simulink library "CH_Library"  (R2021a)
settings: Solver=VariableStepAuto  StartTime=0.0  StopTime=10.0  RelTol=1e-3
undefined symbols (not defined in the file or in its folder): params, X, Y, Z
libraries: sm_lib x116, nesl_utility x53, $bdroot x20, sm_humanoid_walker_lib x13, fl_lib x10, simulink x8, ee_lib x3, simulink_extras x1
(part 1 of 4)
settings Model: Creator=The MathWorks, Inc.  LastModifiedBy=coa19cdd
settings SolverCC: AlgebraicLoopSolver=TrustRegion
settings DebuggingCC: SFMachineParentedDataDiag=warning

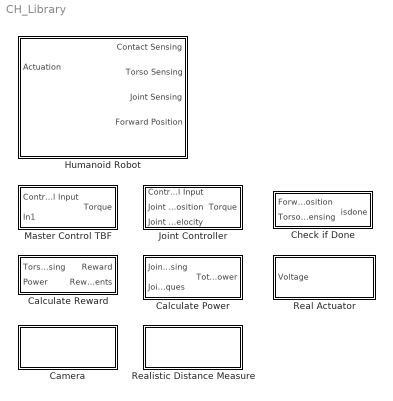
== system CH_Library ==
  Calculate Power : Subsystem
  Calculate Reward : Subsystem  mask{forwardReward=params.reward.forwardRewardWeight, timestepReward=params.reward.timestepRewardWeight, powerPenalty=params.reward.powerPenaltyWeight, verticalPenalty=params.reward.verticalPenaltyWeight, lateralPenalty=params.reward.lateralPenaltyWeight}
      mask prompts: forwardReward "Forward velcoity reward scaling"; timestepReward "Timestep reward scaling"; powerPenalty "Power penalty scaling"; verticalPenalty "Vertical displacement penalty scaling"; lateralPenalty "Lateral displacement penalty scaling"
  Camera : Subsystem  mask{X_ROT=0, Z_ROT=0, X_TF=0, Y_TF=0, Z_TF=0}
      mask prompts: X_ROT "X rotation Value"; Z_ROT "Z Rotation Value"; X_TF "X Displacement"; Y_TF "Y Displacement"; Z_TF "Z Displacement"
      mask DialogControl Container7 Prompt: Camera Rotation
      mask DialogControl Container8 Prompt: Camera Transform
  Check if Done : Subsystem  mask{verticalStop=params.stoppingCriteria.heightChange, lateralStop=params.stoppingCriteria.lateral, angularStop=params.stoppingCriteria.angle, timeoutTime=params.stoppingCriteria.timeoutTime, timeoutDistance=params.stoppingCriteria.timeoutDistance}
      mask prompts: verticalStop "Vertical Displacement Stopping Criteria (m)"; lateralStop "Lateral Displacement Stopping Criteria (m)"; angularStop "Rotation Stopping Criteria (deg)"; timeoutTime "Timeout Time"; timeoutDistance "Timeout Distance"
  Humanoid Robot : Subsystem  mask{contactRadius=params.contact.contactRadius, contactStiffness=params.contact.stiffness, contactDamping=params.contact.damping, contactTWidth=params.contact.transitionWidth, contactStaticFriction=params.contact.staticFriction, contactDynamicFriction=params.contact.dynamicFriction, contactCriticalVelocity=params.contact.criticalVelocity, footDensity=params.materialProperties.lowerBodyDensity, lowerLegDensity=params.materialProperties.lowerBodyDensity, upperLegDensity=params.materialProperties.lowerBodyDensity, hipDensity=params.materialProperties.lowerBodyDensity, trunkDensity=params.materialProperties.upperBodyDensity, shoulderDensity=params.materialProperties.upperBodyDensity, upperArmDensity=params.materialProperties.upperBodyDensity, lowerArmDensity=params.materialProperties.upperBodyDensity, handDensity=params.materialProperties.upperBodyDensity, headDensity=params.materialProperties.upperBodyDensity, hipUpperLimit=params.jointLimits.hipFrontalUpperLimit, hipLowerLimit=params.jointLimits.hipFrontalLowerLimit, kneeUpperLimit=params.jointLimits.kneeUpperLimit, kneeLowerLimit=params.jointLimits.kneeLowerLimit, ankleUpperLimit=params.jointLimits.ankleUpperLimit, ankleLowerLimit=params.jointLimits.ankleLowerLimit, shoulderFrontalUpperLimit=params.jointLimits.shoulderFrontalUpperLimit, shoulderFrontalLowerLimit=params.jointLimits.shoulderFrontalLowerLimit, shoulderSagittalUpperLimit=params.jointLimits.shoulderSagittalUpperLimit, shoulderSagittalLowerLimit=params.jointLimits.shoulderSagittalLowerLimit, elbowUpperLimit=params.jointLimits.ankleUpperLimit, elbowLowerLimit=params.jointLimits.shoulderSagittalLowerLimit, wristUpperLimit=params.jointLimits.ankleUpperLimit, wristLowerLimit=params.jointLimits.shoulderSagittalLowerLimit}
      mask prompts: contactRadius "Contact Sphere Radius (m)"; contactStiffness "Contact Stiffness (N/m)"; contactDamping "Contact Damping (Ns/m)"; contactTWidth "Contact Tranisiton Region Width (m)"; contactStaticFriction "Contact Static Friction"; contactDynamicFriction "Contact Dynamic Friction"; contactCriticalVelocity "Contact Critical Velocity (m/s)"; footDensity "Foot Density (kg/m^3)"; lowerLegDensity "Lower Leg Density (kg/m^3)"; upperLegDensity "Upper Leg Density (kg/m^3)"; hipDensity "Hip Density (kg/m^3)"; trunkDensity "Trunk Density (kg/m^3)"; shoulderDensity "Shoulder Density (kg/m^3)"; upperArmDensity "Upper Arm Density (kg/m^3)"; lowerArmDensity "Lower Arm Density (kg/m^3)"; handDensity "Hand Density (kg/m^3)"; headDensity "Neck / Head Density (kg/m^3)"; hipUpperLimit "Hip Frontal Upper Limit (deg)"; hipLowerLimit "Hip Frontal Lower Limit (deg)"; kneeUpperLimit "Knee Upper Limit (deg)"; kneeLowerLimit "Knee Lower Limit (deg)"; ankleUpperLimit "Ankle Upper Limit (deg)"; ankleLowerLimit "Ankle Lower Limit (deg)"; shoulderFrontalUpperLimit "Shoulder Frontal Upper Limit (deg)"; shoulderFrontalLowerLimit "Shoulder Frontal Lower Limit (deg)"; shoulderSagittalUpperLimit "Shoulder Sagittal Upper Limit (deg)"; shoulderSagittalLowerLimit "Shoulder Sagittal Lower Limit (deg)"; elbowUpperLimit "Elbow Upper Limit (deg)"; elbowLowerLimit "Elbow Lower Limit (deg)"; wristUpperLimit "Wrist Upper Limit (deg)"; wristLowerLimit "Wrist Lower Limit (deg)"
      mask DialogControl Container4 Prompt: Contact Parameters
      mask DialogControl Container9 Prompt: Material Properties
      mask DialogControl Container12 Prompt: Joint Parameters
      mask DialogControl Container10 Prompt: LegLimits
      mask DialogControl Container11 Prompt: ArmLimits
  Joint Controller : Subsystem  mask{jointStiffness=0, jointDamping=0, jointUpperLimit=0, jointLowerLimit=0, jointTorqueLimit=0}
      mask prompts: jointStiffness "Joint Control Stiffness (N*m/rad)"; jointDamping "Joint Control Damping (N*m*s/rad)"; jointUpperLimit "Joint Upper Limit (deg)"; jointLowerLimit "Joint Lower Limt (deg)"; jointTorqueLimit "Joint Absolute Torque Limit (N*m)"
      mask DialogControl DescTextVar Prompt: Stiffness based joint controller.
  Master Control TBF : Subsystem
  Real Actuator : Subsystem  mask{ArmatureInductance=0, StallTorque=0, NoLoadSpeed=0, RatedDCSupply=0, gearRatio=5.0}
      mask prompts: ArmatureInductance "Armature Inductance"; StallTorque "Stall Torque"; NoLoadSpeed "Maximum Speed"; RatedDCSupply "Rated DC Supply Voltage"; gearRatio "Gearing ratio"
      settings: PortSchema="{\"entries\":[{\"content\":{\"sides\":[{\"content\":{\"connectorIds\":[\"In1\"]},\"type\":\"ConnectorPlacement.EquallySpacedRectSide\",\"uuid\":\"1974e72c-7cd0-4a5e-a369-6bd8d81aeaf4\"},{\"content\":{\"connectorIds\":[],\"side\":\"RIGHT\"},\"type\":\"ConnectorPlacement.EquallySpacedRectSide\",\"uuid\":\"85686b63-5bbe-4355-a058-7d010135ed1d\"},{\"content\":{\"connectorIds\":[\"LConn1\",\"LConn2\"],\"side\":\"TOP\"},\"type\":\"ConnectorPlacement.EquallySpacedRectSide\",\"uuid\":\"5bc14ff2-42d4-4faf-9552-836511591ac4\"}]},\"type\":\"ConnectorPlacement.EquallySpacedConnector\",\"uuid\":\"9c3e7e84-92ff-47c5-b2ae-92b3c6517a43\"}],\"packageUris\":[\"http://schema.mathworks.com/mf0/Connector/R2020b\"],\"version\":\"1.0\"}"
      mask DialogControl Container4 Prompt: Motor parameters
      mask DialogControl Container5 Prompt: Gearbox Ratio
  Realistic Distance Measure : Subsystem  mask{LEDC=0.500}
      mask prompts: LEDC "LED Current"

== system CH_Library/Calculate Power ==
  Joint Sensing : Inport
  Joint Torques : Inport  Port=2
  Bus Selector1 : BusSelector  OutputSignals=LegSense.RightLegSense.RHFS.rhThetaDot,LegSense.RightLegSense.RHSS.rhssThetaDot,LegSense.RightLegSense.RKS.rkThetaDot,LegSense.RightLegSense.RAS.raThetaDot,LegSense.RightLegSense.RASS.lasThetaDot,LegSense.LeftLegSense.LHFS.lhThetaDot,LegSense.LeftLegSense.LHSS.lhsThetaDot,LegSense.LeftLegSense.LKS.lkThetaDot,LegSense.LeftLegSense.LASS.lasThetaDot,LegSense.LeftLegSense.LAS.laThetaDot,ArmSense.RightArmSense.RSFS.rsfThetaDot,ArmSense.RightArmSense.RSSS.rssThetaDot,ArmSense.RightArmSense.RES.reThetaDot,ArmSense.RightArmSense.RWS.rwThetaDot,ArmSense.LeftArmSense.LSFS.lsfThetaDot,ArmSense.LeftArmSense.LSSS.lssThetaDot,ArmSense.LeftArmSense.LES.leThetaDot,ArmSense.LeftArmSense.LWS.lwThetaDot
  Mux : Mux  Inputs=18
  Product : Product
  Sum of Elements : Sum  Inputs=+
  Unit Delay : UnitDelay  SampleTime=-1  HasFrameUpgradeWarning=on
  Total Power : Outport
  wires:
  Bus Selector1/18 -> Mux/18  "<lwThetaDot>"
  Bus Selector1/17 -> Mux/17  "<leThetaDot>"
  Bus Selector1/16 -> Mux/16  "<lssThetaDot>"
  Bus Selector1/15 -> Mux/15  "<lsfThetaDot>"
  Bus Selector1/14 -> Mux/14  "<rwThetaDot>"
  Bus Selector1/13 -> Mux/13  "<reThetaDot>"
  Bus Selector1/12 -> Mux/12  "<rssThetaDot>"
  Bus Selector1/11 -> Mux/11  "<rsfThetaDot>"
  Bus Selector1/10 -> Mux/10  "<laThetaDot>"
  Bus Selector1/9 -> Mux/9  "<lasThetaDot>"
  Bus Selector1/8 -> Mux/8  "<lkThetaDot>"
  Bus Selector1/7 -> Mux/7  "<lhsThetaDot>"
  Bus Selector1/6 -> Mux/6  "<lhThetaDot>"
  Bus Selector1/5 -> Mux/5  "<lasThetaDot>"
  Bus Selector1/4 -> Mux/4  "<raThetaDot>"
  Bus Selector1/3 -> Mux/3  "<rkThetaDot>"
  Bus Selector1/2 -> Mux/2  "<rhssThetaDot>"
  Bus Selector1/1 -> Mux/1  "<rhThetaDot>"
  Product/1 -> Sum of Elements/1
  Joint Sensing/1 -> Bus Selector1/1
  Mux/1 -> Product/1
  Joint Torques/1 -> Product/2
  Sum of Elements/1 -> Unit Delay/1
  Unit Delay/1 -> Total Power/1

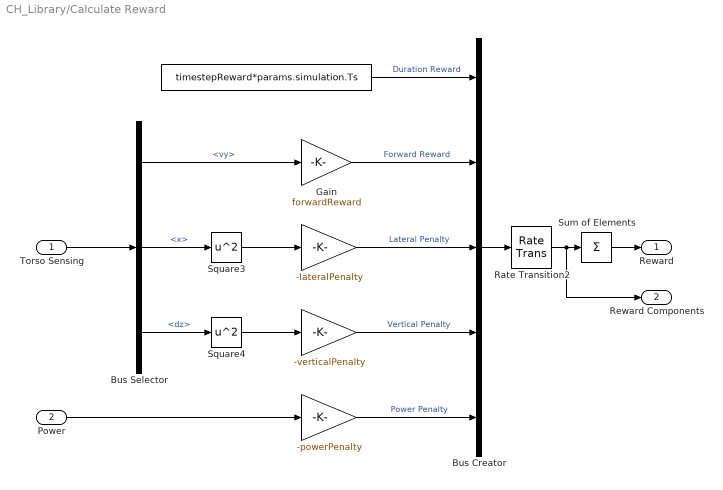
== system CH_Library/Calculate Reward ==
  Torso Sensing : Inport
  Power : Inport  Port=2
  " " : Gain  Gain=-lateralPenalty
  "     " : Gain  Gain=-verticalPenalty
  "                    " : Gain  Gain=-powerPenalty
  "                       " : Constant  Value=timestepReward*params.simulation.Ts
  Bus Creator : BusCreator  Inputs=5
  Bus Selector : BusSelector  OutputSignals=signal2.vy,signal2.x,signal2.dz
  Gain : Gain  Gain=forwardReward
  Rate Transition2 : RateTransition  OutPortSampleTime=params.simulation.Ts
  Square3 : Math  Operator=square  SignedPower=on  SaturateOnIntegerOverflow=on
  Square4 : Math  Operator=square  SignedPower=on  SaturateOnIntegerOverflow=on
  Sum of Elements : Sum  Inputs=+
  Reward : Outport  VectorParamsAs1DForOutWhenUnconnected=off
  Reward Components : Outport  Port=2  VectorParamsAs1DForOutWhenUnconnected=off
  wires:
  Torso Sensing/1 -> Bus Selector/1
  Power/1 -> "                    "/1
  Square4/1 -> "     "/1
  Bus Selector/3 -> Square4/1  "<dz>"
  Square3/1 -> " "/1
  Bus Selector/2 -> Square3/1  "<x>"
  Sum of Elements/1 -> Reward/1
  " "/1 -> Bus Creator/3  "Lateral Penalty"
  "                    "/1 -> Bus Creator/5  "Power Penalty"
  "                       "/1 -> Bus Creator/1  "Duration Reward"
  Bus Selector/1 -> Gain/1  "<vy>"
  Gain/1 -> Bus Creator/2  "Forward Reward"
  "     "/1 -> Bus Creator/4  "Vertical Penalty"
  Bus Creator/1 -> Rate Transition2/1
  Rate Transition2/1 -> Reward Components/1, Sum of Elements/1

== system CH_Library/Camera ==
  Camera Location : sm_lib/Frames and Transforms/Rigid Transform  TranslationMethod=Cartesian  TranslationStandardOffset=0  TranslationLengthUnit=m  TranslationStandardAxis=+Z  TranslationCartesianOffset=[X_TF Y_TF Z_TF]  TranslationROffset=0  TranslationROffsetUnits=m  TranslationZOffset=0  TranslationZOffsetUnits=m  TranslationThetaOffset=0  TranslationThetaOffsetUnits=deg  RotationMethod=None  RotationAngleUnits=deg  RotationStandardAxis=+Z  RotationAngle=0.0  RotationArbitraryAxis=[0 0 1]  FollAlignAxisA=+X  BaseAlignAxisA=+Y  FollAlignAxisB=+Y  BaseAlignAxisB=+Z  RotationSequenceAxes=FollowerAxes  RotationSequence=XYX  RotationSequenceAngles=[0 0 0]  RotationSequenceAnglesUnits=deg  RotationMatrix=[1 0 0; 0 1 0; 0 0 1]
  Camera Rotation : sm_lib/Frames and Transforms/Rigid Transform  TranslationMethod=None  TranslationStandardOffset=0  TranslationLengthUnit=m  TranslationStandardAxis=+Z  TranslationCartesianOffset=[0 0 0]  TranslationROffset=0  TranslationROffsetUnits=m  TranslationZOffset=0  TranslationZOffsetUnits=m  TranslationThetaOffset=0  TranslationThetaOffsetUnits=deg  RotationMethod=RotationSequence  RotationAngleUnits=deg  RotationStandardAxis=+Z  RotationAngle=0.0  RotationArbitraryAxis=[0 0 1]  FollAlignAxisA=+X  BaseAlignAxisA=+Y  FollAlignAxisB=+Y  BaseAlignAxisB=+Z  RotationSequenceAxes=FollowerAxes  RotationSequence=ZXZ  RotationSequenceAngles=[Z_ROT X_ROT 0]  RotationSequenceAnglesUnits=deg  RotationMatrix=[1 0 0; 0 1 0; 0 0 1]
  Spherical Solid : sm_lib/Body Elements/Spherical Solid  GraphicAmbientColor=[0.15 0.15 0.15 1.0]  BasedOnType=Density  CenterOfMass=[0 0 0]  CenterOfMassUnits=m  GraphicDiffuseColor=[0.2 1.0 0.2]  Density=1000  DensityUnits=kg/m^3  DoExposeReferenceFrame=on  GraphicEmissiveColor=[0.0 0.0 0.0 1.0]  ExportEntireGeometry=off  SerializedExposedGeometries=<ExposedGeometries/>  SerializedFrames=<Frames/>  MarkerShape=Sphere  MarkerSize=10  GraphicType=FromGeometry  InertiaType=PointMass  Mass=1  MassUnits=g  MomentsOfInertia=[1 1 1]  MomentsOfInertiaUnits=kg*m^2  GraphicOpacity=1.0  ProductsOfInertia=[0 0 0]  ProductsOfInertiaUnits=kg*m^2  GraphicShininess=75  GraphicSpecularColor=[0.5 0.5 0.5 1.0]  SphereRadius=0.01  SphereRadiusUnits=m  GraphicVisPropType=SimpleVisualProperties
  Camera : PMIOPort  Side=Right
  connections:
  Spherical Solid/RConn1 -- Camera Location/RConn1
  Camera Rotation/RConn1 -- Camera Location/LConn1
  Camera/RConn1 -- Camera Rotation/LConn1

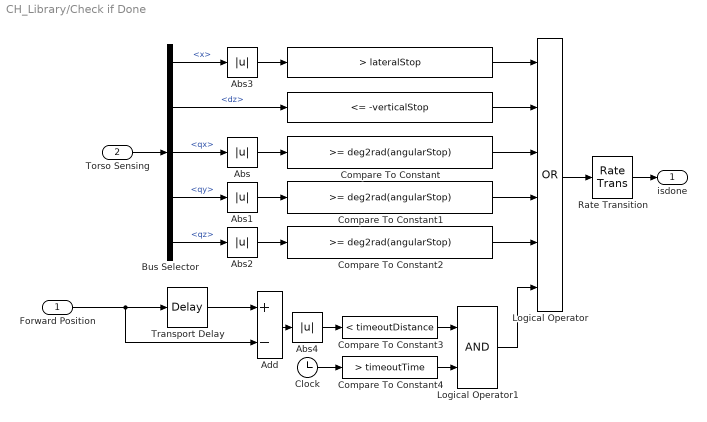
== system CH_Library/Check if Done ==
  Forward Position : Inport
  Torso Sensing : Inport  Port=2
  " " : simulink/Logic and Bit Operations/Compare To Constant  relop=<=  const=-verticalStop  OutDataTypeStr=boolean  ZeroCross=off
  "             " : simulink/Logic and Bit Operations/Compare To Constant  relop=>  const=lateralStop  OutDataTypeStr=boolean
  Abs{,1..3} (4 alike) : Abs  ZeroCross=off
  Abs4 : Abs
  Add : Sum  Inputs=+-
  Bus Selector : BusSelector  OutputSignals=signal2.x,signal2.dz,signal1.qx,signal1.qy,signal1.qz
  Clock : Clock
  Compare To Constant : simulink/Logic and Bit Operations/Compare To Constant  relop=>=  const=deg2rad(angularStop)  OutDataTypeStr=boolean  ZeroCross=off
  Compare To Constant1 : simulink/Logic and Bit Operations/Compare To Constant  relop=>=  const=deg2rad(angularStop)  OutDataTypeStr=boolean  ZeroCross=off
  Compare To Constant2 : simulink/Logic and Bit Operations/Compare To Constant  relop=>=  const=deg2rad(angularStop)  OutDataTypeStr=boolean  ZeroCross=off
  Compare To Constant3 : simulink/Logic and Bit Operations/Compare To Constant  relop=<  const=timeoutDistance  OutDataTypeStr=boolean
  Compare To Constant4 : simulink/Logic and Bit Operations/Compare To Constant  relop=>  const=timeoutTime  OutDataTypeStr=boolean
  Logical Operator : Logic  Operator=OR  Inputs=6  AllPortsSameDT=off  OutDataTypeStr=boolean
  Logical Operator1 : Logic  AllPortsSameDT=off  OutDataTypeStr=boolean
  Rate Transition : RateTransition  OutPortSampleTime=params.simulation.Ts
  Transport Delay : TransportDelay  DelayTime=timeoutTime  BufferSize=8192
  isdone : Outport  VectorParamsAs1DForOutWhenUnconnected=off
  wires:
  Bus Selector/2 -> " "/1  "<dz>"
  Torso Sensing/1 -> Bus Selector/1
  " "/1 -> Logical Operator/2
  Bus Selector/3 -> Abs/1  "<qx>"
  Bus Selector/4 -> Abs1/1  "<qy>"
  Compare To Constant/1 -> Logical Operator/3
  Abs/1 -> Compare To Constant/1
  Abs1/1 -> Compare To Constant1/1
  Logical Operator/1 -> Rate Transition/1
  Abs3/1 -> "             "/1
  Bus Selector/1 -> Abs3/1  "<x>"
  "             "/1 -> Logical Operator/1
  Abs2/1 -> Compare To Constant2/1
  Bus Selector/5 -> Abs2/1  "<qz>"
  Compare To Constant2/1 -> Logical Operator/5
  Compare To Constant1/1 -> Logical Operator/4
  Rate Transition/1 -> isdone/1
  Forward Position/1 -> Add/2, Transport Delay/1
  Transport Delay/1 -> Add/1
  Add/1 -> Abs4/1
  Abs4/1 -> Compare To Constant3/1
  Clock/1 -> Compare To Constant4/1
  Logical Operator1/1 -> Logical Operator/6
  Compare To Constant3/1 -> Logical Operator1/1
  Compare To Constant4/1 -> Logical Operator1/2

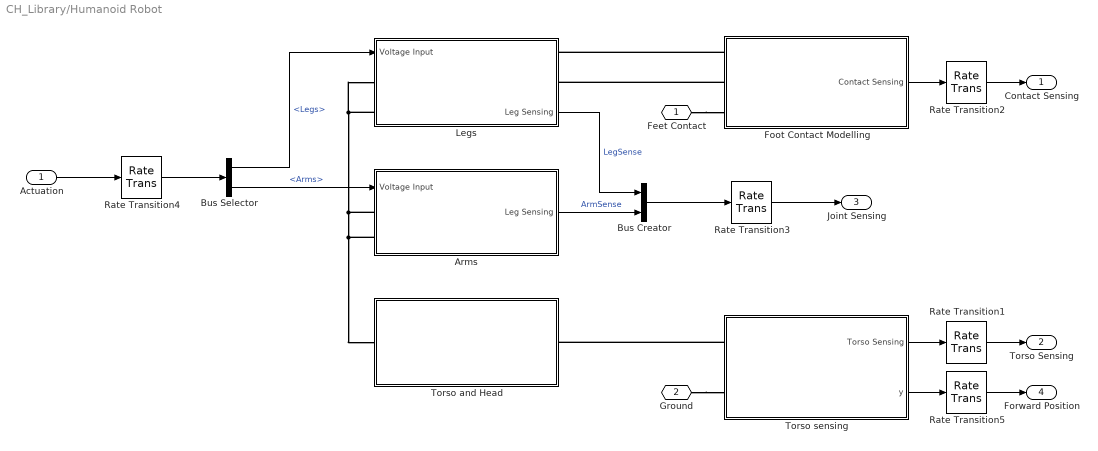
== system CH_Library/Humanoid Robot ==
  Actuation : Inport
  Arms : Subsystem
  Bus Creator : BusCreator  Inputs=2
  Bus Selector : BusSelector  OutputSignals=Legs,Arms
  Foot Contact Modelling : Subsystem
  Legs : Subsystem
      settings: PortSchema="{\"entries\":[{\"content\":{\"sides\":[{\"content\":{\"connectorIds\":[\"In1\",\"LConn1\",\"LConn2\"]},\"type\":\"ConnectorPlacement.EquallySpacedRectSide\",\"uuid\":\"23351413-746b-4a06-be1b-12a3513cfbfe\"},{\"content\":{\"connectorIds\":[\"RConn1\",\"RConn2\",\"Out1\"],\"side\":\"RIGHT\"},\"type\":\"ConnectorPlacement.EquallySpacedRectSide\",\"uuid\":\"11cf50da-2174-4e1a-8294-03a32c066ee9\"},{\"content\":{\"connectorIds\":[],\"side\":\"TOP\"},\"type\":\"ConnectorPlacement.EquallySpacedRectSide\",\"uuid\":\"131464a5-eb41-49e4-a10b-6e29adf56ddb\"}]},\"type\":\"ConnectorPlacement.EquallySpacedConnector\",\"uuid\":\"d1829b9e-a701-4b79-9220-5146acc6850e\"}],\"packageUris\":[\"http://schema.mathworks.com/mf0/Connector/R2020b\"],\"version\":\"1.0\"}"
  Rate Transition{1..5} (5 alike) : RateTransition  OutPortSampleTime=params.simulation.Ts
  Torso and Head : Subsystem
  Torso sensing : Subsystem
  Feet Contact : PMIOPort  Side=Right
  " Ground" : PMIOPort  Port=2  Side=Left
  Contact Sensing : Outport
  Torso Sensing : Outport  Port=2
  Joint Sensing : Outport  Port=3
  Forward Position : Outport  Port=4
  wires:
  Foot Contact Modelling/1(Contact Sensing) -> Rate Transition2/1
  Actuation/1 -> Rate Transition4/1
  Torso sensing/1(Torso Sensing) -> Rate Transition1/1
  Rate Transition2/1 -> Contact Sensing/1
  Rate Transition1/1 -> Torso Sensing/1
  Rate Transition3/1 -> Joint Sensing/1
  Rate Transition5/1 -> Forward Position/1
  Torso sensing/2(y) -> Rate Transition5/1
  Rate Transition4/1 -> Bus Selector/1
  Bus Selector/1 -> Legs/1(Voltage Input)  "<Legs>"
  Bus Selector/2 -> Arms/1(Voltage Input)  "<Arms>"
  Bus Creator/1 -> Rate Transition3/1
  Legs/1(Leg Sensing) -> Bus Creator/1  "LegSense"
  Arms/1(Leg Sensing) -> Bus Creator/2  "ArmSense"
  connections:
  Legs/LConn2 -- Legs/LConn1 -- Arms/LConn1 -- Arms/LConn2 -- Torso and Head/LConn1
  Torso sensing/LConn1 -- Torso and Head/RConn1
  Feet Contact/RConn1 -- Foot Contact Modelling/LConn3
  Foot Contact Modelling/LConn1 -- Legs/RConn1
  Foot Contact Modelling/LConn2 -- Legs/RConn2
  " Ground"/RConn1 -- Torso sensing/LConn2

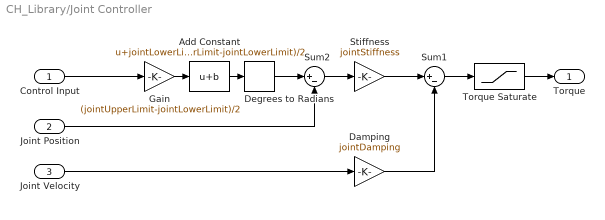
== system CH_Library/Joint Controller ==
  Control Input : Inport
  Joint Position : Inport  Port=2
  Joint Velocity : Inport  Port=3
  Add Constant : Bias  Bias=jointLowerLimit + (jointUpperLimit-jointLowerLimit)/2
  Damping : Gain  Gain=jointDamping
  Degrees to Radians : simulink_extras/Transformations/Degrees to Radians
  Gain : Gain  Gain=(jointUpperLimit-jointLowerLimit)/2
  Stiffness : Gain  Gain=jointStiffness
  Sum1 : Sum  Inputs=|+-
  Sum2 : Sum  Inputs=|+-
  Torque Saturate : Saturate  UpperLimit=jointTorqueLimit  LowerLimit=-jointTorqueLimit  ZeroCross=off
  Torque : Outport
  wires:
  Damping/1 -> Sum1/2
  Stiffness/1 -> Sum1/1
  Add Constant/1 -> Degrees to Radians/1
  Gain/1 -> Add Constant/1
  Control Input/1 -> Gain/1
  Sum2/1 -> Stiffness/1
  Joint Velocity/1 -> Damping/1
  Sum1/1 -> Torque Saturate/1
  Torque Saturate/1 -> Torque/1
  Degrees to Radians/1 -> Sum2/1
  Joint Position/1 -> Sum2/2

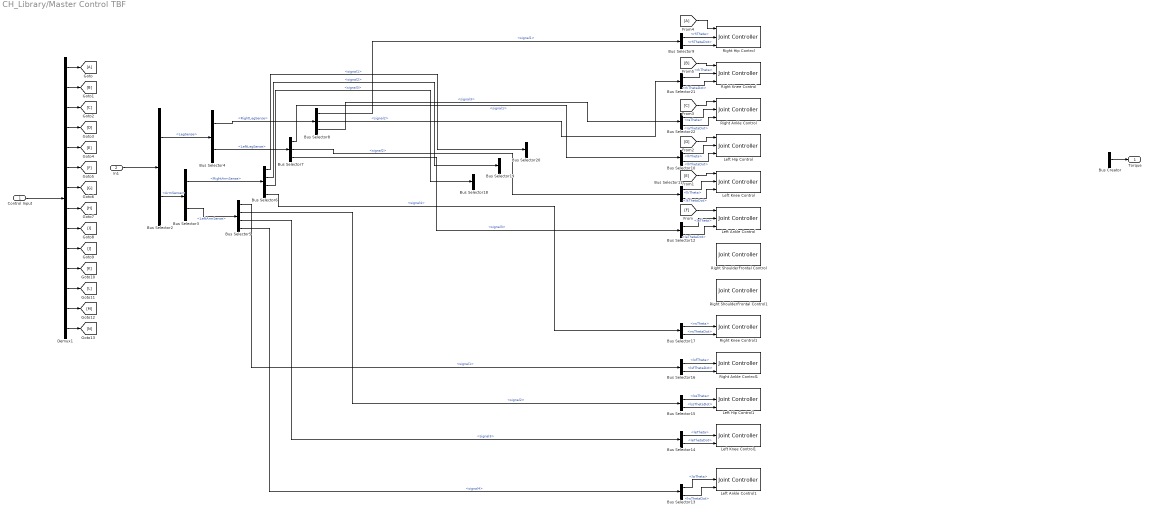
== system CH_Library/Master Control TBF ==
  Control Input : Inport
  In1 : Inport  Port=2
  Bus Creator : BusCreator  Inputs=2
  Bus Selector10 : BusSelector  OutputSignals=lhTheta,lhThetaDot
  Bus Selector11 : BusSelector  OutputSignals=lkTheta,lkThetaDot
  Bus Selector12 : BusSelector  OutputSignals=laTheta,laThetaDot
  Bus Selector13 : BusSelector  OutputSignals=lwTheta,lwThetaDot
  Bus Selector14 : BusSelector  OutputSignals=leTheta,leThetaDot
  Bus Selector15 : BusSelector  OutputSignals=lssTheta,lssThetaDot
  Bus Selector16 : BusSelector  OutputSignals=lsfTheta,lsfThetaDot
  Bus Selector17 : BusSelector  OutputSignals=rwTheta,rwThetaDot
  Bus Selector18 : BusSelector  OutputSignals=reTheta,reThetaDot
  Bus Selector19 : BusSelector  OutputSignals=rssTheta,rssThetaDot
  Bus Selector2 : BusSelector  OutputSignals=LegSense,ArmSense
  Bus Selector20 : BusSelector  OutputSignals=rsfTheta,rsfThetaDot
  Bus Selector21 : BusSelector  OutputSignals=rkTheta,rkThetaDot
  Bus Selector22 : BusSelector  OutputSignals=raTheta,raThetaDot
  Bus Selector3 : BusSelector  OutputSignals=RightArmSense,LeftArmSense
  Bus Selector4 : BusSelector  OutputSignals=RightLegSense,LeftLegSense
  Bus Selector5 : BusSelector  OutputSignals=signal1,signal2,signal3,signal4
  Bus Selector6 : BusSelector  OutputSignals=signal1,signal2,signal3,signal4
  Bus Selector7 : BusSelector  OutputSignals=signal1,signal2,signal3
  Bus Selector8 : BusSelector  OutputSignals=signal1,signal2,signal3
  Bus Selector9 : BusSelector  OutputSignals=rhTheta,rhThetaDot
  Demux1 : Demux  Outputs=14
  Left Ankle Control : sm_humanoid_walker_lib/Joint Controller  jointStiffness=params.controller.ankleStiffness  jointDamping=params.controller.ankleDamping  jointUpperLimit=params.jointLimits.ankleUpperLimit  jointLowerLimit=params.jointLimits.ankleLowerLimit  jointTorqueLimit=params.torqueLimits.ankle
  Left Ankle Control1 : sm_humanoid_walker_lib/Joint Controller  jointStiffness=params.controller.ankleStiffness  jointDamping=params.controller.ankleDamping  jointUpperLimit=params.jointLimits.ankleUpperLimit  jointLowerLimit=params.jointLimits.ankleLowerLimit  jointTorqueLimit=params.torqueLimits.ankle
  Left Hip Control : sm_humanoid_walker_lib/Joint Controller  jointStiffness=params.controller.hipFrontalStiffness  jointDamping=params.controller.hipFrontalDamping  jointUpperLimit=params.jointLimits.hipFrontalUpperLimit  jointLowerLimit=params.jointLimits.hipFrontalLowerLimit  jointTorqueLimit=params.torqueLimits.hipFrontal
  Left Hip Control1 : sm_humanoid_walker_lib/Joint Controller  jointStiffness=params.controller.hipFrontalStiffness  jointDamping=params.controller.hipFrontalDamping  jointUpperLimit=params.jointLimits.hipFrontalUpperLimit  jointLowerLimit=params.jointLimits.hipFrontalLowerLimit  jointTorqueLimit=params.torqueLimits.hipFrontal
  Left Knee Control : sm_humanoid_walker_lib/Joint Controller  jointStiffness=params.controller.kneeStiffness  jointDamping=params.controller.kneeDamping  jointUpperLimit=params.jointLimits.kneeUpperLimit  jointLowerLimit=params.jointLimits.kneeLowerLimit  jointTorqueLimit=params.torqueLimits.knee
  Left Knee Control1 : sm_humanoid_walker_lib/Joint Controller  jointStiffness=params.controller.kneeStiffness  jointDamping=params.controller.kneeDamping  jointUpperLimit=params.jointLimits.kneeUpperLimit  jointLowerLimit=params.jointLimits.kneeLowerLimit  jointTorqueLimit=params.torqueLimits.knee
  Right Ankle Control : sm_humanoid_walker_lib/Joint Controller  jointStiffness=params.controller.ankleStiffness  jointDamping=params.controller.ankleDamping  jointUpperLimit=params.jointLimits.ankleUpperLimit  jointLowerLimit=params.jointLimits.ankleLowerLimit  jointTorqueLimit=params.torqueLimits.ankle
  Right Ankle Control1 : sm_humanoid_walker_lib/Joint Controller  jointStiffness=params.controller.ankleStiffness  jointDamping=params.controller.ankleDamping  jointUpperLimit=params.jointLimits.ankleUpperLimit  jointLowerLimit=params.jointLimits.ankleLowerLimit  jointTorqueLimit=params.torqueLimits.ankle
  Right Hip Control : sm_humanoid_walker_lib/Joint Controller  jointStiffness=params.controller.hipFrontalStiffness  jointDamping=params.controller.hipFrontalDamping  jointUpperLimit=params.jointLimits.hipFrontalUpperLimit  jointLowerLimit=params.jointLimits.hipFrontalLowerLimit  jointTorqueLimit=params.torqueLimits.hipFrontal
  Right Knee Control : sm_humanoid_walker_lib/Joint Controller  jointStiffness=params.controller.kneeStiffness  jointDamping=params.controller.kneeDamping  jointUpperLimit=params.jointLimits.kneeUpperLimit  jointLowerLimit=params.jointLimits.kneeLowerLimit  jointTorqueLimit=params.torqueLimits.knee
  Right Knee Control1 : sm_humanoid_walker_lib/Joint Controller  jointStiffness=params.controller.kneeStiffness  jointDamping=params.controller.kneeDamping  jointUpperLimit=params.jointLimits.kneeUpperLimit  jointLowerLimit=params.jointLimits.kneeLowerLimit  jointTorqueLimit=params.torqueLimits.knee
  Right ShoulderFrontal Control : sm_humanoid_walker_lib/Joint Controller  jointStiffness=params.controller.hipFrontalStiffness  jointDamping=params.controller.hipFrontalDamping  jointUpperLimit=params.jointLimits.shoulderFrontalUpperLimit  jointLowerLimit=params.jointLimits.shoulderFrontalLowerLimit  jointTorqueLimit=params.torqueLimits.hipFrontal
  Right ShoulderFrontal Control1 : sm_humanoid_walker_lib/Joint Controller  jointStiffness=params.controller.hipFrontalStiffness  jointDamping=params.controller.hipFrontalDamping  jointUpperLimit=params.jointLimits.shoulderFrontalUpperLimit  jointLowerLimit=params.jointLimits.shoulderFrontalLowerLimit  jointTorqueLimit=params.torqueLimits.hipFrontal
  Torque : Outport
  wires:
  Control Input/1 -> Demux1/1
  Demux1/1 -> [A]
  Demux1/6 -> [F]
  Demux1/5 -> [E]
  Demux1/4 -> [D]
  Demux1/3 -> [C]
  Demux1/2 -> [B]
  [F] -> Left Ankle Control/1
  [E] -> Left Knee Control/1
  [D] -> Left Hip Control/1
  [C] -> Right Ankle Control/1
  [B] -> Right Knee Control/1
  Demux1/7 -> [G]
  Demux1/8 -> [H]
  Demux1/9 -> [I]
  Demux1/10 -> [J]
  Demux1/11 -> [K]
  Demux1/12 -> [L]
  Bus Creator/1 -> Torque/1
  ? -> Bus Creator/1
  Demux1/13 -> [M]
  Demux1/14 -> [N]
  Bus Selector7/2 -> Bus Selector11/1  "<signal2>"
  Bus Selector6/1 -> Bus Selector20/1  "<signal1>"
  Bus Selector4/2 -> Bus Selector7/1  "<LeftLegSense>"
  Bus Selector8/3 -> Bus Selector22/1  "<signal3>"
  Bus Selector8/1 -> Bus Selector9/1  "<signal1>"
  Bus Selector3/1 -> Bus Selector6/1  "<RightArmSense>"
  Bus Selector2/2 -> Bus Selector3/1  "<ArmSense>"
  Bus Selector7/1 -> Bus Selector10/1  "<signal1>"
  Bus Selector7/3 -> Bus Selector12/1  "<signal3>"
  In1/1 -> Bus Selector2/1
  Bus Selector8/2 -> Bus Selector21/1  "<signal2>"
  Bus Selector4/1 -> Bus Selector8/1  "<RightLegSense>"
  Bus Selector5/3 -> Bus Selector14/1  "<signal3>"
  Bus Selector6/2 -> Bus Selector19/1  "<signal2>"
  Bus Selector3/2 -> Bus Selector5/1  "<LeftArmSense>"
  Bus Selector5/4 -> Bus Selector13/1  "<signal4>"
  Bus Selector5/1 -> Bus Selector16/1  "<signal1>"
  Bus Selector6/4 -> Bus Selector17/1  "<signal4>"
  Bus Selector5/2 -> Bus Selector15/1  "<signal2>"
  Bus Selector6/3 -> Bus Selector18/1  "<signal3>"
  Bus Selector2/1 -> Bus Selector4/1  "<LegSense>"
  Bus Selector9/1 -> Right Hip Control/2  "<rhTheta>"
  Bus Selector9/2 -> Right Hip Control/3  "<rhThetaDot>"
  [A] -> Right Hip Control/1
  Bus Selector21/1 -> Right Knee Control/2  "<rkTheta>"
  Bus Selector21/2 -> Right Knee Control/3  "<rkThetaDot>"
  Bus Selector22/1 -> Right Ankle Control/2  "<raTheta>"
  Bus Selector22/2 -> Right Ankle Control/3  "<raThetaDot>"
  Bus Selector10/1 -> Left Hip Control/2  "<lhTheta>"
  Bus Selector10/2 -> Left Hip Control/3  "<lhThetaDot>"
  Bus Selector11/1 -> Left Knee Control/2  "<lkTheta>"
  Bus Selector11/2 -> Left Knee Control/3  "<lkThetaDot>"
  Bus Selector12/1 -> Left Ankle Control/2  "<laTheta>"
  Bus Selector12/2 -> Left Ankle Control/3  "<laThetaDot>"
  Bus Selector13/2 -> Left Ankle Control1/3  "<lwThetaDot>"
  Bus Selector13/1 -> Left Ankle Control1/2  "<lwTheta>"
  Bus Selector14/1 -> Left Knee Control1/2  "<leTheta>"
  Bus Selector14/2 -> Left Knee Control1/3  "<leThetaDot>"
  Bus Selector15/2 -> Left Hip Control1/3  "<lssThetaDot>"
  Bus Selector15/1 -> Left Hip Control1/2  "<lssTheta>"
  Bus Selector16/1 -> Right Ankle Control1/2  "<lsfTheta>"
  Bus Selector16/2 -> Right Ankle Control1/3  "<lsfThetaDot>"
  Bus Selector17/2 -> Right Knee Control1/3  "<rwThetaDot>"
  Bus Selector17/1 -> Right Knee Control1/2  "<rwTheta>"

== system CH_Library/Real Actuator ==
  Voltage : Inport
  Controlled Voltage Source : fl_lib/Electrical/Electrical Sources/Controlled Voltage Source
  DC Motor : ee_lib/Electromechanical/Brushed Motors/DC Motor  field_option=ee.enum.field_option.pm  Rf=100 Ohm  Lf=1 H  Laf=0.15 H  If0=0 A  parameterization=ee.enum.dcparam_option.torque_speed  Ra=3.9 Ohm  La=ArmatureInductance H  emf_or_torque=ee.enum.emf_or_torque.ki  Kv=0.072e-3 V/rpm  Ki=6.876e-4 N*m/A  T_stall=StallTorque N*m  w_max="NoLoadSpeed   rpm"  w_rated=15000 rpm  P_rated=0.08 W  V_rated=RatedDCSupply V  J=0.01 g*cm^2  lam_param=ee.enum.lam_param.damping  lam=0 N*m/(rad/s)  i_noload=0 A  V_i_noload=1.5 V  speed0=0 rpm  enable_fault_armature=ee.enum.faults.faultEnable.no  rev_faulted=1 / 3  G_faulted_armature=1e-5 S  fault_trigger_armature=ee.enum.faults.faultTrigger.behavioral  t_fault_armature=1 s  max_permissible_current_armature=4 A  t_fail_on_current_armature=1 s  enable_fault_field=ee.enum.faults.faultEnable.no  G_faulted_field=1e-5 S  fault_trigger_field=ee.enum.faults.faultTrigger.temporal  t_fault_field=1 s  max_permissible_current_field=inf A  t_fail_on_current_field=1 s  fault_action=ee.enum.faults.faultAction.none  alpha=3.93e-3 1/K  Tmeas=25 degC  thermal_mass=100 J/K  initial_temperature=25 degC
  Electrical Reference : fl_lib/Electrical/Electrical Elements/Electrical Reference
  Gear Box : fl_lib/Mechanical/Mechanisms/Gear Box  ratio=gearRatio  t_in_specify=off  t_in_priority=None  t_in=0 N*m  t_in_nominal_specify=off  t_in_nominal_unit=N*m  t_in_nominal_value=1  t_out_specify=off  t_out_priority=None  t_out=0 N*m  t_out_nominal_specify=off  t_out_nominal_unit=N*m  t_out_nominal_value=1
  Mechanical Rotational Reference : fl_lib/Mechanical/Rotational Elements/Mechanical Rotational Reference
  Rotational Multibody Interface1 : fl_lib/Mechanical/Multibody Interfaces/Rotational Multibody Interface
      settings: SourceProductBaseCode=SS
  Simulink-PS Converter : nesl_utility/Simulink-PS Converter  PhysicalDomain=network_engine_domain  SubClassName=ps_input  LeftPortType=input  RightPortType=output  PseudoPeriodic=off  Frequencies=[]  NoiseDistribution=none  NoiseParameters=[]  Unit=1  AffineConversion=off  FilteringAndDerivatives=provide  SimscapeFilterOrder=1  InputFilterTimeConstant=0.001  UdotUserProvided=0
      settings: SourceProductBaseCode=PW,SS
  T : PMIOPort  Side=Left
  W : PMIOPort  Port=2  Side=Left
  wires:
  Voltage/1 -> Simulink-PS Converter/1
  connections:
  Rotational Multibody Interface1/RConn1 -- W/RConn1
  Rotational Multibody Interface1/LConn1 -- T/RConn1
  Simulink-PS Converter/RConn1 -- Controlled Voltage Source/RConn1
  Controlled Voltage Source/RConn2 -- DC Motor/LConn1
  Controlled Voltage Source/LConn1 -- DC Motor/RConn1 -- Electrical Reference/LConn1
  DC Motor/LConn2 -- Gear Box/LConn1
  DC Motor/RConn2 -- Rotational Multibody Interface1/RConn2 -- Mechanical Rotational Reference/LConn1
  Gear Box/RConn1 -- Rotational Multibody Interface1/LConn2

== system CH_Library/Realistic Distance Measure ==
  note: https://cdn.shopify.com/s/files/1/0080/8940/3450/files/4052899962101-product-datasheet.pdf?v=14319000425807391721
  note: set distance between robot and object as distance + object radius.
      | Then; if robot is touching object, light will be at it's brightest.
  note: Could cheese distance by having voltage proportional to distance
      | fundamentally the LED needs to plug into the photodiode; Distance would be represented via light intensity of LED rather than actual distance
      |
      | Usable; not preferable
  DC Current Source : fl_lib/Electrical/Electrical Sources/DC Current Source  i0=LEDC A
      settings: SourceProductBaseCode=SS  InternalSimscapePortConfiguration="{\"Bottom\":[],\"Left\":[{\"id\":\"p\",\"label\":\"\",\"type\":\"foundation.electrical.electrical\"}],\"Right\":[{\"id\":\"n\",\"label\":\"\",\"type\":\"foundation.electrical.electrical\"}],\"Top\":[]}"
  Dist^2 : fl_lib/Physical Signals/Functions/PS Math Function  fcn_choice=foundation.enum.math_function.square  v=1
      settings: SourceProductBaseCode=SS
  Electrical Reference : fl_lib/Electrical/Electrical Elements/Electrical Reference
  Electrical Reference1 : fl_lib/Electrical/Electrical Elements/Electrical Reference
  Light-Emitting Diode : ee_lib/Sensors & Transducers/Light-Emitting Diode  Gain=0.005 W/A  prmExp=1  I12=[.0017, .003] A  V12=[.9, 1.05] V  IS=5e-5 A  ec=10  RS=0.1 Ohm  Tmeas=25 degC  C_param=1  CJ=20 pF  CJ0=20 pF  VJ=1 V  Mgrad=0.5  Vvec=[.1, 10, 100] V  Cvec=[15, 10, 2] pF  FC=0.5  T_param=1  IS_T2=1.8e-4 A  I1_T2=0.0034 A  V1_T2=1.05 V  Tmeas2=125 degC  EG_param=1  EG=1.11 eV  XTI_param=1  XTI=3  Tdevice=25 degC  i_capacitor_specify=off  i_capacitor_priority=High  i_capacitor=0 A  i_capacitor_nominal_specify=off  i_capacitor_nominal_unit=A  i_capacitor_nominal_value=1  v_capacitor_specify=off  v_capacitor_priority=None  v_capacitor=0 V  v_capacitor_nominal_specify=off  v_capacitor_nominal_unit=V  v_capacitor_nominal_value=1  thermal_network_parameterization=ee.enum.thermalNetworkTopology.cauer  Rth=[0, 10] K/W  Rth_Foster=[4, 6] K/W  thermal_mass_parameterization=ee.enum.thermalNetwork.timeconstant  thermal_mass=[0, 1] J/K  thermal_mass_Foster=[1.5, 3] J/K  thermal_time_constant=[0, 10] s  thermal_time_constant_Foster=[6, 18] s  thermal_mass_initial_temperatures=[25, 25] degC
      settings: SourceProductBaseCode=PS  InternalSimscapePortConfiguration="{\"Bottom\":[],\"Left\":[{\"id\":\"W\",\"label\":\"W\",\"type\":\"output\"},{\"id\":\"p\",\"label\":\"\",\"type\":\"foundation.electrical.electrical\"}],\"Right\":[{\"id\":\"n\",\"label\":\"\",\"type\":\"foundation.electrical.electrical\"}],\"Top\":[]}"
  Lux/dist^2 : fl_lib/Physical Signals/Functions/PS Divide
      settings: SourceProductBaseCode=SS
  Photodiode : ee_lib/Sensors & Transducers/Photodiode  prmFlux=2  Imeas=25 uA  FluxD=5 W/m^2  G=5e-6 m^2*A/W  prmExp=2  I2=0.1 A  V2=1.3 V  IS=5e-9 A  ec=3  RS=0.1 Ohm  Tmeas=25 degC  C_param=1  CJ=60 pF  CJ0=60 pF  VJ=1 V  Mgrad=0.5  Vvec=[.1, 10, 100] V  Cvec=[45, 3, 6] pF  FC=0.5  T_param=1  IS_T2=2.5e-7 A  I1_T2=0.07 A  V1_T2=1.3 V  Tmeas2=125 degC  EG_param=1  EG=1.11 eV  XTI_param=1  XTI=3  Tdevice=25 degC  i_capacitor_specify=off  i_capacitor_priority=High  i_capacitor=0 A  i_capacitor_nominal_specify=off  i_capacitor_nominal_unit=A  i_capacitor_nominal_value=1  v_capacitor_specify=off  v_capacitor_priority=None  v_capacitor=0 V  v_capacitor_nominal_specify=off  v_capacitor_nominal_unit=V  v_capacitor_nominal_value=1  thermal_network_parameterization=ee.enum.thermalNetworkTopology.cauer  Rth=[0, 10] K/W  Rth_Foster=[4, 6] K/W  thermal_mass_parameterization=ee.enum.thermalNetwork.timeconstant  thermal_mass=[0, 1] J/K  thermal_mass_Foster=[1.5, 3] J/K  thermal_time_constant=[0, 10] s  thermal_time_constant_Foster=[6, 18] s  thermal_mass_initial_temperatures=[25, 25] degC
      settings: SourceProductBaseCode=PS  InternalSimscapePortConfiguration="{\"Bottom\":[],\"Left\":[{\"id\":\"W\",\"label\":\"W\",\"type\":\"input\"},{\"id\":\"p\",\"label\":\"\",\"type\":\"foundation.electrical.electrical\"}],\"Right\":[{\"id\":\"n\",\"label\":\"\",\"type\":\"foundation.electrical.electrical\"}],\"Top\":[]}"
  Transform Sensor : sm_lib/Frames and Transforms/Transform Sensor  MeasurementFrame=Base  SenseAngle=off  SenseAxis=off  SenseAngle1=off  SenseAngle2=off  SenseAngle3=off  SenseQ=off  SenseR=off  SenseOmegaX=off  SenseOmegaY=off  SenseOmegaZ=off  SenseOmega1=off  SenseOmega2=off  SenseOmega3=off  SenseQDot=off  SenseRDot=off  SenseAlphaX=off  SenseAlphaY=off  SenseAlphaZ=off  SenseAlpha1=off  SenseAlpha2=off  SenseAlpha3=off  SenseQDDot=off  SenseRDDot=off  SenseX=off  SenseY=off  SenseZ=off  SenseRad=off  SenseAzim=off  SenseDist=on  SenseInc=off  SenseXDot=off  SenseYDot=off  SenseZDot=off  SenseRadDot=off  SenseAzimDot=off  SenseDistDot=off  SenseIncDot=off  SenseXDDot=off  SenseYDDot=off  SenseZDDot=off  SenseRadDDot=off  SenseAzimDDot=off  SenseDistDDot=off  SenseIncDDot=off
  Input Frame : PMIOPort  Side=Left
  Output Frame : PMIOPort  Port=2  Side=Right
  Output Voltage : PMIOPort  Port=3  Side=Right
  connections:
  Lux/dist^2/LConn1 -- Light-Emitting Diode/LConn1
  Photodiode/LConn1 -- Lux/dist^2/RConn1
  Dist^2/RConn1 -- Lux/dist^2/LConn2
  Transform Sensor/RConn2 -- Dist^2/LConn1
  Transform Sensor/LConn1 -- Input Frame/RConn1
  Output Frame/RConn1 -- Transform Sensor/RConn1
  Output Voltage/RConn1 -- Photodiode/RConn1
  Electrical Reference/LConn1 -- Light-Emitting Diode/LConn2 -- DC Current Source/RConn1
  Electrical Reference1/LConn1 -- Photodiode/LConn2
  DC Current Source/LConn1 -- Light-Emitting Diode/RConn1

== system CH_Library/Humanoid Robot/Arms ==
  Voltage Input : Inport
  Bus Creator1 : BusCreator  Inputs=2
  Bus Selector : BusSelector  OutputSignals=RightArm,LeftArm
  Left Arm : Subsystem
  Right Arm : Subsystem
  Right Shoulder : PMIOPort  Side=Left
  Left Shoulder : PMIOPort  Port=2  Side=Left
  Leg Sensing : Outport
  wires:
  Bus Selector/2 -> Left Arm/1(Voltage Input)  "<LeftArm>"
  Bus Selector/1 -> Right Arm/1(Voltage Input)  "<RightArm>"
  Voltage Input/1 -> Bus Selector/1
  Left Arm/1(Sensing) -> Bus Creator1/2
  Right Arm/1(Sensing) -> Bus Creator1/1
  Bus Creator1/1 -> Leg Sensing/1
  connections:
  Right Arm/LConn1 -- Right Shoulder/RConn1
  Left Arm/LConn1 -- Left Shoulder/RConn1

== system CH_Library/Humanoid Robot/Foot Contact Modelling ==
  Bus Creator : BusCreator  Inputs=2
  Left Foot Contact : $bdroot/Humanoid Robot/Foot Contact Modelling/Right Foot Contact  SystemSampleTime=-1  VariantActivationTime=update diagram  Latency=0  AutoFrameSizeCalculation=off
  Right Foot Contact : Subsystem
  Right Foot Contact Points : PMIOPort  Side=Left
  Left Foot Contact Points : PMIOPort  Port=2  Side=Left
  Feet Contact : PMIOPort  Port=3  Side=Left
  Contact Sensing : Outport
  wires:
  Left Foot Contact/1 -> Bus Creator/2  "leftContact"
  Right Foot Contact/1(Foot Force) -> Bus Creator/1  "rightContact"
  Bus Creator/1 -> Contact Sensing/1
  connections:
  Right Foot Contact/LConn1 -- Right Foot Contact Points/RConn1
  Right Foot Contact/RConn1 -- Left Foot Contact/RConn1 -- Feet Contact/RConn1
  Left Foot Contact/LConn1 -- Left Foot Contact Points/RConn1

== system CH_Library/Humanoid Robot/Legs ==
  Voltage Input : Inport
  Bus Creator1 : BusCreator  Inputs=2
  Bus Selector : BusSelector  OutputSignals=RightLeg,LeftLeg
  Left Leg : Subsystem
  Right leg : Subsystem
  Right Hip : PMIOPort  Side=Left
  Left Hip : PMIOPort  Port=2  Side=Left
  Right Foot : PMIOPort  Port=3  Side=Right
  Left Foot : PMIOPort  Port=4  Side=Right
  Leg Sensing : Outport
  wires:
  Bus Selector/1 -> Right leg/1(Torque Input)  "<RightLeg>"
  Bus Selector/2 -> Left Leg/1(Torque Input)  "<LeftLeg>"
  Voltage Input/1 -> Bus Selector/1
  Left Leg/1(Sensing) -> Bus Creator1/2
  Right leg/1(Sensing) -> Bus Creator1/1
  Bus Creator1/1 -> Leg Sensing/1
  connections:
  Left Hip/RConn1 -- Left Leg/LConn1
  Right Foot/RConn1 -- Right leg/RConn1
  Left Foot/RConn1 -- Left Leg/RConn1
  Right Hip/RConn1 -- Right leg/LConn1

== system CH_Library/Humanoid Robot/Torso and Head ==
  Camera : $bdroot/Camera  X_ROT=0  Z_ROT=0  X_TF=0  Y_TF=0  Z_TF=0
  Cover : sm_lib/Body Elements/File Solid  ExtGeomFileName=sm_humanoid_walker_cover.stp  UnitType=FromFile  ExtGeomFileUnits=m  StepReaderType=HEX  ExportConvexHullGeometry=off  InertiaType=CalculateFromGeometry  Mass=0  MassUnits=kg  CenterOfMass=[0, 0, 0]  CenterOfMassUnits=m  MomentsOfInertia=[0, 0, 0]  MomentsOfInertiaUnits=kg*m^2  ProductsOfInertia=[0, 0, 0]  ProductsOfInertiaUnits=kg*m^2  BasedOnType=Density  Density=headDensity  DensityUnits=kg/m^3  DoExposeReferenceFrame=on  SerializedFrames=<Frames/>  GraphicType=FromGeometry  MarkerShape=Sphere  MarkerSize=10  GraphicVisPropType=SimpleVisualProperties  GraphicDiffuseColor=[1, 1, 1]  GraphicSpecularColor=[0.5 0.5 0.5 1.0]  GraphicAmbientColor=[0.15 0.15 0.15 1.0]  GraphicEmissiveColor=[0.0 0.0 0.0 1.0]  GraphicShininess=75  GraphicOpacity=1
  Head : sm_lib/Body Elements/File Solid  ExtGeomFileName=sm_humanoid_walker_head.stp  UnitType=FromFile  ExtGeomFileUnits=m  StepReaderType=HEX  ExportConvexHullGeometry=off  InertiaType=CalculateFromGeometry  Mass=0  MassUnits=kg  CenterOfMass=[0, 0, 0]  CenterOfMassUnits=m  MomentsOfInertia=[0, 0, 0]  MomentsOfInertiaUnits=kg*m^2  ProductsOfInertia=[0, 0, 0]  ProductsOfInertiaUnits=kg*m^2  BasedOnType=Density  Density=headDensity  DensityUnits=kg/m^3  DoExposeReferenceFrame=on  SerializedFrames=<Frames/>  GraphicType=FromGeometry  MarkerShape=Sphere  MarkerSize=10  GraphicVisPropType=SimpleVisualProperties  GraphicDiffuseColor=[0.0 0.0 0.0]  GraphicSpecularColor=[0.5 0.5 0.5 1.0]  GraphicAmbientColor=[0.15 0.15 0.15 1.0]  GraphicEmissiveColor=[0.0 0.0 0.0 1.0]  GraphicShininess=75  GraphicOpacity=1
  Head Origin Transformation : sm_lib/Frames and Transforms/Rigid Transform  TranslationMethod=Cartesian  TranslationStandardOffset=0  TranslationLengthUnit=m  TranslationStandardAxis=+Z  TranslationCartesianOffset=[0, 0, 0.06414]*3.5  TranslationROffset=0  TranslationROffsetUnits=m  TranslationZOffset=0  TranslationZOffsetUnits=m  TranslationThetaOffset=0  TranslationThetaOffsetUnits=deg  RotationMethod=RotationSequence  RotationAngleUnits=deg  RotationStandardAxis=+Z  RotationAngle=0.0  RotationArbitraryAxis=[0 0 1]  FollAlignAxisA=+X  BaseAlignAxisA=+Y  FollAlignAxisB=+Y  BaseAlignAxisB=+Z  RotationSequenceAxes=BaseAxes  RotationSequence=XYZ  RotationSequenceAngles=[0, 0, 0]  RotationSequenceAnglesUnits=rad  RotationMatrix=[1 0 0; 0 1 0; 0 0 1]
  Neck : sm_lib/Body Elements/File Solid  ExtGeomFileName=sm_humanoid_walker_neck.stp  UnitType=FromFile  ExtGeomFileUnits=m  StepReaderType=HEX  ExportConvexHullGeometry=off  InertiaType=CalculateFromGeometry  Mass=0  MassUnits=kg  CenterOfMass=[0, 0, 0]  CenterOfMassUnits=m  MomentsOfInertia=[0, 0, 0]  MomentsOfInertiaUnits=kg*m^2  ProductsOfInertia=[0, 0, 0]  ProductsOfInertiaUnits=kg*m^2  BasedOnType=Density  Density=headDensity  DensityUnits=kg/m^3  DoExposeReferenceFrame=on  SerializedFrames=<Frames/>  GraphicType=FromGeometry  MarkerShape=Sphere  MarkerSize=10  GraphicVisPropType=SimpleVisualProperties  GraphicDiffuseColor=[0.0 0.0 0.0]  GraphicSpecularColor=[0.5 0.5 0.5 1.0]  GraphicAmbientColor=[0.15 0.15 0.15 1.0]  GraphicEmissiveColor=[0.0 0.0 0.0 1.0]  GraphicShininess=75  GraphicOpacity=1
  Neck Origin Tranformation : sm_lib/Frames and Transforms/Rigid Transform  TranslationMethod=Cartesian  TranslationStandardOffset=0  TranslationLengthUnit=m  TranslationStandardAxis=+Z  TranslationCartesianOffset=[0, 0, 0.01016]*3.5  TranslationROffset=0  TranslationROffsetUnits=m  TranslationZOffset=0  TranslationZOffsetUnits=m  TranslationThetaOffset=0  TranslationThetaOffsetUnits=deg  RotationMethod=RotationSequence  RotationAngleUnits=deg  RotationStandardAxis=+Z  RotationAngle=0.0  RotationArbitraryAxis=[0 0 1]  FollAlignAxisA=+X  BaseAlignAxisA=+Y  FollAlignAxisB=+Y  BaseAlignAxisB=+Z  RotationSequenceAxes=BaseAxes  RotationSequence=XYZ  RotationSequenceAngles=[0, 0, 0]  RotationSequenceAnglesUnits=rad  RotationMatrix=[1 0 0; 0 1 0; 0 0 1]
  Shoulder : sm_lib/Body Elements/File Solid  ExtGeomFileName=sm_humanoid_walker_shoulder.stp  UnitType=FromFile  ExtGeomFileUnits=m  StepReaderType=HEX  ExportConvexHullGeometry=off  InertiaType=CalculateFromGeometry  Mass=0  MassUnits=kg  CenterOfMass=[0, 0, 0]  CenterOfMassUnits=m  MomentsOfInertia=[0, 0, 0]  MomentsOfInertiaUnits=kg*m^2  ProductsOfInertia=[0, 0, 0]  ProductsOfInertiaUnits=kg*m^2  BasedOnType=Density  Density=shoulderDensity  DensityUnits=kg/m^3  DoExposeReferenceFrame=on  SerializedFrames=<Frames/>  GraphicType=FromGeometry  MarkerShape=Sphere  MarkerSize=10  GraphicVisPropType=SimpleVisualProperties  GraphicDiffuseColor=[1.0 0.6 0.6]  GraphicSpecularColor=[0.5 0.5 0.5 1.0]  GraphicAmbientColor=[0.15 0.15 0.15 1.0]  GraphicEmissiveColor=[0.0 0.0 0.0 1.0]  GraphicShininess=75  GraphicOpacity=1
  Shoulder Origin Transformation : sm_lib/Frames and Transforms/Rigid Transform  TranslationMethod=Cartesian  TranslationStandardOffset=0  TranslationLengthUnit=m  TranslationStandardAxis=+Z  TranslationCartesianOffset=[0, 0, -0.0399]*3.5  TranslationROffset=0  TranslationROffsetUnits=m  TranslationZOffset=0  TranslationZOffsetUnits=m  TranslationThetaOffset=0  TranslationThetaOffsetUnits=deg  RotationMethod=RotationSequence  RotationAngleUnits=deg  RotationStandardAxis=+Z  RotationAngle=0.0  RotationArbitraryAxis=[0 0 1]  FollAlignAxisA=+X  BaseAlignAxisA=+Y  FollAlignAxisB=+Y  BaseAlignAxisB=+Z  RotationSequenceAxes=BaseAxes  RotationSequence=XYZ  RotationSequenceAngles=[0, 0, 0]  RotationSequenceAnglesUnits=rad  RotationMatrix=[1 0 0; 0 1 0; 0 0 1]
  Trunk : sm_lib/Body Elements/File Solid  ExtGeomFileName=sm_humanoid_walker_trunk.stp  UnitType=FromFile  ExtGeomFileUnits=km  StepReaderType=HEX  ExportConvexHullGeometry=off  InertiaType=CalculateFromGeometry  Mass=0  MassUnits=kg  CenterOfMass=[0, 0, 0]  CenterOfMassUnits=m  MomentsOfInertia=[0, 0, 0]  MomentsOfInertiaUnits=kg*m^2  ProductsOfInertia=[0, 0, 0]  ProductsOfInertiaUnits=kg*m^2  BasedOnType=Density  Density=trunkDensity  DensityUnits=kg/m^3  DoExposeReferenceFrame=on  SerializedFrames=<Frames/>  GraphicType=FromGeometry  MarkerShape=Sphere  MarkerSize=10  GraphicVisPropType=SimpleVisualProperties  GraphicDiffuseColor=[1.0 0.2 0.2]  GraphicSpecularColor=[0.5 0.5 0.5 1.0]  GraphicAmbientColor=[0.15 0.15 0.15 1.0]  GraphicEmissiveColor=[0.0 0.0 0.0 1.0]  GraphicShininess=75  GraphicOpacity=1
  Torso : PMIOPort  Side=Left
  Torso Ref : PMIOPort  Port=2  Side=Right
  connections:
  Shoulder Origin Transformation/LConn1 -- Torso Ref/RConn1 -- Torso/RConn1 -- Trunk/RConn1
  Head/RConn1 -- Camera/RConn1 -- Cover/RConn1 -- Head Origin Transformation/RConn1
  Shoulder/RConn1 -- Shoulder Origin Transformation/RConn1 -- Neck Origin Tranformation/LConn1
  Neck Origin Tranformation/RConn1 -- Head Origin Transformation/LConn1 -- Neck/RConn1
